simulink model "IK_SG_simulation"  (R2023a)
settings: Solver=VariableStepAuto  StartTime=0.0  StopTime=34  RelTol=1e-3
libraries: simulink x2
settings Model: Creator=Ahmed Sedky  LastModifiedBy=Ahmed Sedky

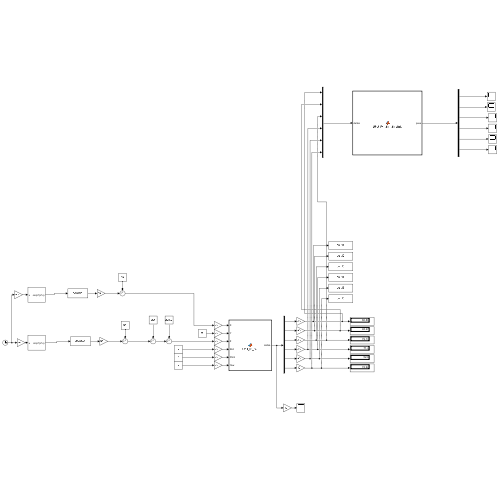
[thumbnail: Simulink's stored preview of the top-level diagram]
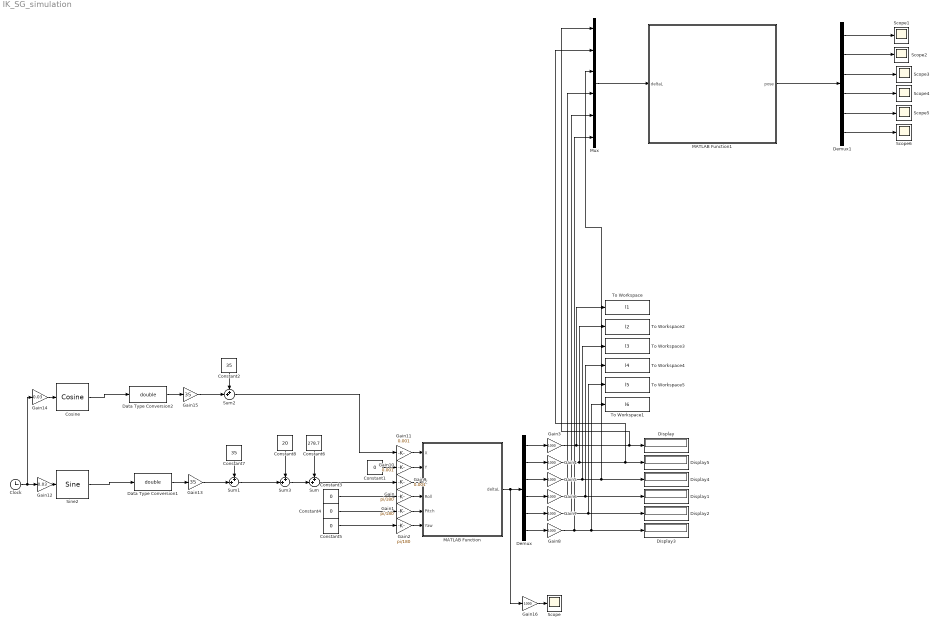
== system IK_SG_simulation ==
  Clock : Clock
  Constant{1,3..5} (4 alike) : Constant  Value=0
  Constant2 : Constant  Value=35
  Constant6 : Constant  Value=278.7
  Constant7 : Constant  Value=35
  Constant8 : Constant  Value=20
  Cosine : simulink/Lookup Tables/Cosine  Formula=cos(2*pi*u)  NumDataPoints=(2^5)+1  OutputWordLength=16  InternalRulePriority=Speed
  Data Type Conversion1 : DataTypeConversion  OutDataTypeStr=double  SaturateOnIntegerOverflow=off  RndMeth=Floor
  Data Type Conversion2 : DataTypeConversion  OutDataTypeStr=double  SaturateOnIntegerOverflow=off  RndMeth=Floor
  Demux : Demux  Outputs=6
  Demux1 : Demux  Outputs=6
  Display{,1..5} (6 alike) : Display
  Gain : Gain  Gain=pi/180
  Gain1 : Gain  Gain=pi/180
  Gain10 : Gain  Gain=0.001
  Gain11 : Gain  Gain=0.001
  Gain12 : Gain  Gain=0.03
  Gain13 : Gain  Gain=35
  Gain14 : Gain  Gain=0.03
  Gain15 : Gain  Gain=35
  Gain{3..8,16} (7 alike) : Gain  Gain=1000
  Gain2 : Gain  Gain=pi/180
  Gain9 : Gain  Gain=0.001
  MATLAB Function : MATLAB Function  TreatAsAtomicUnit=on
  MATLAB Function1 : MATLAB Function  TreatAsAtomicUnit=on
  Mux : Mux  Inputs=6
  Scope{,1..6} (7 alike) : Scope
  Sine2 : simulink/Lookup Tables/Sine  Formula=sin(2*pi*u)  NumDataPoints=(2^5)+1  OutputWordLength=16  InternalRulePriority=Speed
  Sum{,1..3} (4 alike) : Sum  Inputs=++|
  To Workspace : ToWorkspace  VariableName=l1  SaveFormat=Timeseries  SampleTime=0.01
  To Workspace1 : ToWorkspace  VariableName=l6  SaveFormat=Timeseries  SampleTime=0.01
  To Workspace2 : ToWorkspace  VariableName=l2  SaveFormat=Timeseries  SampleTime=0.01
  To Workspace3 : ToWorkspace  VariableName=l3  SaveFormat=Timeseries  SampleTime=0.01
  To Workspace4 : ToWorkspace  VariableName=l4  SaveFormat=Timeseries  SampleTime=0.01
  To Workspace5 : ToWorkspace  VariableName=l5  SaveFormat=Timeseries  SampleTime=0.01
  wires:
  MATLAB Function/1(deltaL) -> Gain16/1, Demux/1
  Gain2/1 -> MATLAB Function/6(Yaw)
  Gain1/1 -> MATLAB Function/5(Pitch)
  Gain/1 -> MATLAB Function/4(Roll)
  Sum2/1 -> Gain11/1
  Sum/1 -> Gain9/1
  Constant1/1 -> Gain10/1
  Constant3/1 -> Gain/1
  Constant4/1 -> Gain1/1
  Constant5/1 -> Gain2/1
  Demux/1 -> Gain3/1
  Demux/5 -> Gain7/1
  Demux/6 -> Gain8/1
  Demux/4 -> Gain6/1
  Demux/3 -> Gain5/1
  Demux/2 -> Gain4/1
  Gain3/1 -> To Workspace/1, Mux/1, Display/1
  Gain4/1 -> To Workspace2/1, Mux/2, Display5/1
  Gain5/1 -> To Workspace3/1, Mux/3, Display4/1
  Gain6/1 -> Mux/4, To Workspace4/1, Display1/1
  Gain7/1 -> Mux/5, To Workspace5/1, Display2/1
  Gain8/1 -> Mux/6, To Workspace1/1, Display3/1
  Constant6/1 -> Sum/1
  Sum1/1 -> Sum3/2
  Gain11/1 -> MATLAB Function/1(X)
  Gain10/1 -> MATLAB Function/2(Y)
  Gain9/1 -> MATLAB Function/3(Z)
  Gain13/1 -> Sum1/2
  Gain12/1 -> Sine2/1
  Clock/1 -> Gain14/1, Gain12/1
  Sine2/1 -> Data Type Conversion1/1
  Constant7/1 -> Sum1/1
  Data Type Conversion1/1 -> Gain13/1
  Cosine/1 -> Data Type Conversion2/1
  Gain14/1 -> Cosine/1
  Constant2/1 -> Sum2/1
  Data Type Conversion2/1 -> Gain15/1
  Gain15/1 -> Sum2/2
  Sum3/1 -> Sum/2
  Constant8/1 -> Sum3/1
  Gain16/1 -> Scope/1
  Mux/1 -> MATLAB Function1/1(deltaL)
  MATLAB Function1/1(pose) -> Demux1/1
  Demux1/1 -> Scope1/1
  Demux1/2 -> Scope2/1
  Demux1/3 -> Scope3/1
  Demux1/4 -> Scope4/1
  Demux1/5 -> Scope5/1
  Demux1/6 -> Scope6/1

== matlab function IK_SG_simulation/MATLAB Function1 ==
  data: deltaL input; pose output
function pose = UPU_FK_Sim_Simulink(deltaL)
%#codegen
% Simulink-compatible Forward Kinematics (Newton-Raphson)
% Input : deltaL(6x1)
% Output: pose(6x1) = [X Y Z Roll Pitch Yaw]

%% --- Geometry Definition ---
Rb = 0.185; Rp = 0.150; l0 = 0.29;

angleB = deg2rad([25 49 145 169 265 289]);
angleP = deg2rad([0 74 120 194 240 314]);

b = zeros(3,6);
p = zeros(3,6);
for i = 1:6
    b(:,i) = [Rb*cos(angleB(i)); Rb*sin(angleB(i)); 0];
    p(:,i) = [Rp*cos(angleP(i)); Rp*sin(angleP(i)); 0];
end

l_measured = l0 + deltaL(:);

%% --- Initial Guess ---
x = [0; 0; 0.29; 0; 0; 0];

%% --- Iterative Solver ---
for k = 1:20   % Max 20 iterations
    [F, J] = legLengthErrorAndJacobian(x, b, p, l_measured);
    dx = -J\F;
    x = x + dx;
    if norm(dx) < 1e-6
        break;
    end
end

pose = x;  % [X Y Z Roll Pitch Yaw]
end

%% --- Helper Function ---
function [F, J] = legLengthErrorAndJacobian(x, b, p, l_measured)
X = x(1); Y = x(2); Z = x(3);
Roll = x(4); Pitch = x(5); Yaw = x(6);

cy = cos(Yaw); sy = sin(Yaw);
cp = cos(Pitch); sp = sin(Pitch);
cr = cos(Roll); sr = sin(Roll);

R = [cy*cp, cy*sp*sr - sy*cr, cy*sp*cr + sy*sr;
     sy*cp, sy*sp*sr + cy*cr, sy*sp*cr - cy*sr;
     -sp,   cp*sr,            cp*cr];

r = [X; Y; Z];
F = zeros(6,1);
J = zeros(6,6);

for i = 1:6
    L = r + R*p(:,i) - b(:,i);
    l = norm(L);
    F(i) = l - l_measured(i);
    % Jacobian rows: dL/d[X Y Z Roll Pitch Yaw]
    if l == 0
        continue;
    end
    u = L / l;
    % Partial derivatives wrt position
    J(i,1:3) = u';
    % Partial wrt rotation (approx small-angle Jacobian)
    dpdR = cross(u, R*p(:,i))';
    J(i,4:6) = dpdR;
end
end

== matlab function IK_SG_simulation/MATLAB Function ==
  data: X input; deltaL output; Y input; Z input; Roll input; Pitch input; Yaw input
function deltaL = UPU_IK_Sim(X, Y, Z, Roll, Pitch, Yaw)
%#codegen
% UPU_IK_Sim: Inverse Kinematics for UPU Stewart Platform
%
% Inputs : X, Y, Z         -> translation of platform center [m]
%          Roll, Pitch, Yaw -> rotation angles [rad]
% Output : deltaL(6x1)     -> leg length changes from home [m]
%
% Geometry parameters and base/platform layout defined internally.
% Home length l0 = 0.4 m

%% --- Geometry Definition ---
Rb = 0.185;   % Base radius [m]
Rp = 0.150;  % Platform radius [m]
l0 = 0.29;   % Nominal leg length [m]

% Joint angle layout (hexagonal)
angleB = deg2rad([25 49 145 169 265 289]);
angleP = deg2rad([0 74 120 194 240 314]);

b = zeros(3,6);
p = zeros(3,6);
for i = 1:6
    b(:,i) = [Rb*cos(angleB(i)); Rb*sin(angleB(i)); 0];
    p(:,i) = [Rp*cos(angleP(i)); Rp*sin(angleP(i)); 0];
end

%% --- Desired Pose ---
r = [X; Y; Z]; % translation vector

% Rotation matrix (ZYX order: yaw-pitch-roll)
cy = cos(Yaw); sy = sin(Yaw);
cp = cos(Pitch); sp = sin(Pitch);
cr = cos(Roll); sr = sin(Roll);

R = [cy*cp, cy*sp*sr - sy*cr, cy*sp*cr + sy*sr;
     sy*cp, sy*sp*sr + cy*cr, sy*sp*cr - cy*sr;
     -sp,   cp*sr,            cp*cr];

%% --- Compute Leg Lengths ---
l = zeros(1,6);
for i = 1:6
    L = r + R*p(:,i) - b(:,i);
    l(i) = sqrt(L(1)^2 + L(2)^2 + L(3)^2);
end

%% --- Compute Delta Lengths ---
deltaL = (l - l0)';   % column vector [Δl1..Δl6]
end
